simulink model "Cycleconverter"  (R2020a)
settings: Solver=VariableStepDiscrete  StartTime=0.0  StopTime=0.1  RelTol=1e-3
libraries: powerlib x17
settings Model: Creator=Naeem Mohammad  LastModifiedBy=Naeem Mohammad

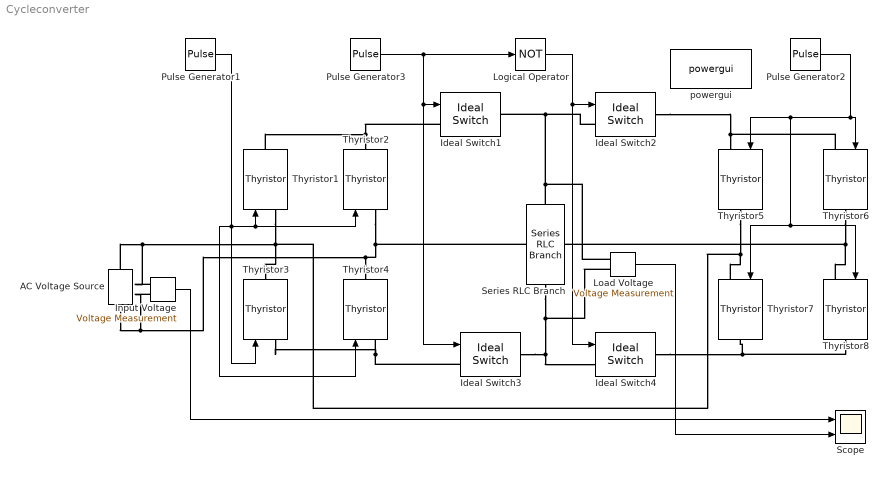
== system Cycleconverter ==
  AC Voltage Source : powerlib/Electrical Sources/AC Voltage Source  Amplitude=220  Phase=0  Frequency=60  SampleTime=0  Measurements=None  BusType=swing  Pref=10e3  Qref=0  Qmin=-inf  Qmax=+inf
  Ideal Switch{1..4} (4 alike) : powerlib/Power Electronics/Ideal Switch  Ron=0.001  Lon=0  IC=0  Rs=1e5  Cs=inf  Measurements=off
  Input Voltage : powerlib/Measurements/Voltage Measurement  PhasorSimulation=off  OutputType=Complex  PSBequivalent=0
  Load Voltage : powerlib/Measurements/Voltage Measurement  PhasorSimulation=off  OutputType=Complex  PSBequivalent=0
  Logical Operator : Logic  Operator=NOT  AllPortsSameDT=off  OutDataTypeStr=boolean
  Pulse Generator1 : DiscretePulseGenerator  PulseType=Time based  Period=0.00835  PulseWidth=50
  Pulse Generator2 : DiscretePulseGenerator  PulseType=Time based  Period=0.00835  PulseWidth=50
  Pulse Generator3 : DiscretePulseGenerator  PulseType=Time based  Period=0.0334  PulseWidth=50
  Scope : Scope  NumInputPorts=2
  Series RLC Branch : powerlib/Elements/Series RLC Branch  LConnTagsString=__new0  RConnTagsString=__new0  BranchType=R  Resistance=1  Inductance=1e-3  SetiL0=off  InitialCurrent=0  Capacitance=1e-6  Setx0=off  InitialVoltage=0  Measurements=None
  Thyristor{1..8} (8 alike) : powerlib/Power Electronics/Thyristor  Ron=0.001  Lon=0  Vf=0.8  IC=0  Rs=500  Cs=250e-9  Measurements=off
  powergui : powerlib/powergui  Priority=1  SimulationMode=Discrete  SampleTime=50e-6  frequency=60  Iterations=50  frequencyindice=60  Pbase=100e6  ErrMax=1e-4  UnitsV=kV  UnitsW=MW  buscounter=0  FunctionMessages=off  echomessages=off  EnableUseOfTLC=off  CurrentSourceSwitches=off  DisableSnubberDevices=off  DisableRonSwitches=off  DisableVfSwitches=off  DisplayEquations=off  AutomaticDiscreteSolvers=off  SolverType=Tustin/Backward Euler (TBE)  Interpol=off  ExternalGateDelay=off  methode=off  Ts=100  x0status=blocks  SPID=on  SwTol=0  HookPort=off  NonlinearTolerance=1e-4  nMaxIteration=100  ContinueOnMaxIteration=off  RestoreLinks=warning  ResistiveCurrentMeasurement=off  Frange=[0:2:500]  Ylog=off  Xlog=on  ShowGrid=off  save=off  variable=ZData  structure=0  ZoomFFT=off  StartTime=0.0  cycles=1  DisplayStyle=1  fundamental=60  FreqAxis=off  MaxFrequency=1000  frequencyindicesteady=1  RmsSteady=1  display=off
  wires:
  Pulse Generator1/1 -> Thyristor2/1, Thyristor1/1, Thyristor4/1, Thyristor3/1
  Pulse Generator2/1 -> Thyristor8/1, Thyristor7/1, Thyristor5/1, Thyristor6/1
  Pulse Generator3/1 -> Logical Operator/1, Ideal Switch3/1, Ideal Switch1/1
  Logical Operator/1 -> Ideal Switch2/1, Ideal Switch4/1
  Input Voltage/1 -> Scope/1
  Load Voltage/1 -> Scope/2
  connections:
  Thyristor1/RConn1 -- Ideal Switch1/LConn1 -- Thyristor2/RConn1
  Thyristor1/LConn1 -- Thyristor5/RConn1 -- Thyristor7/LConn1 -- AC Voltage Source/RConn1 -- Input Voltage/LConn1 -- Thyristor3/RConn1
  Thyristor2/LConn1 -- Thyristor6/RConn1 -- Thyristor8/LConn1 -- Thyristor4/RConn1 -- AC Voltage Source/LConn1 -- Input Voltage/LConn2
  Thyristor3/LConn1 -- Ideal Switch3/LConn1 -- Thyristor4/LConn1
  Series RLC Branch/LConn1 -- Ideal Switch1/RConn1 -- Ideal Switch2/LConn1 -- Load Voltage/LConn1
  Thyristor6/LConn1 -- Ideal Switch2/RConn1 -- Thyristor5/LConn1
  Thyristor8/RConn1 -- Thyristor7/RConn1 -- Ideal Switch4/RConn1
  Ideal Switch3/RConn1 -- Load Voltage/LConn2 -- Series RLC Branch/RConn1 -- Ideal Switch4/LConn1
